simulink model "solution_1"  (R2016a)
settings: Solver=VariableStepAuto  StartTime=0.0  StopTime=10  RelTol=1e-3
undefined symbols (not defined in the file): doppler, fdesignblkfcn, gcbh, startfcn_spectrum_analyzer
libraries: commchan3 x6, dspsrcs4 x5, commrflib2 x5, commanapbnd3 x4, dspsigops x4, commdigbbndpm3 x4, commrandsrc3 x3, dspmtrx3 x1, commanabbnd3 x1, dspfdesign x1, dspspect3 x1, commutil2 x1
settings Model: Creator=Schala  LastModifiedBy=Schala

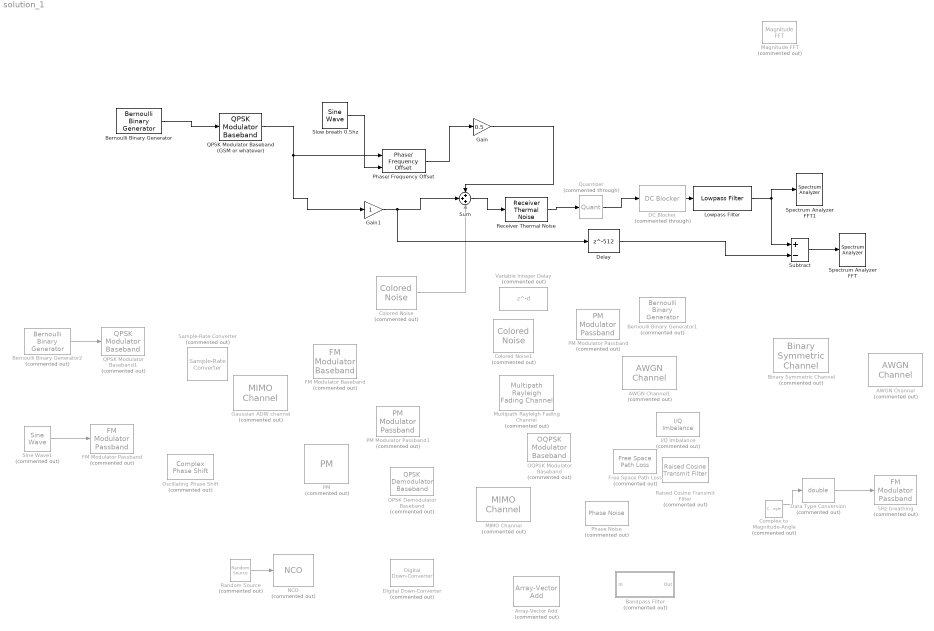
== system solution_1 ==
  "5Hz breathing " : commanapbnd3/FM Modulator Passband  Commented=on  Fc=5  Ph=0  Kc=66
  AWGN Channel : commchan3/AWGN Channel  Commented=on  InputProcessing=Columns as channels (frame based)  seed=67  noiseMode="Signal to noise ratio  (Eb/No)"  EbNodB=10  EsNodB=10  SNRdB=10  bitsPerSym=1  Ps=1  Tsym=1  variance=1
  AWGN Channel1 : commchan3/AWGN Channel  Commented=on  InputProcessing=Columns as channels (frame based)  seed=67  noiseMode="Signal to noise ratio  (Eb/No)"  EbNodB=10  EsNodB=10  SNRdB=10  bitsPerSym=1  Ps=1  Tsym=1  variance=1
  Array-Vector Add : dspmtrx3/Array-Vector Add  Commented=on  Dimension=1  V_Source=Input port  V_VectFromMask=[0.5 0.25]  firstCoeffSignedness=Auto  firstCoeffDataTypeStr=Inherit: Same word length as input  firstCoeffLastDataTypeStr=Inherit: Same word length as input  firstCoeffMin=[]  firstCoeffMax=[]  outputSignedness=Auto  outputDataTypeStr=Inherit: Same as accumulator  outputLastDataTypeStr=Inherit: Same as accumulator  outputMin=[]  outputMax=[]  accumSignedness=Auto  prodOutputSignedness=Auto  roundingMode=Floor  overflowMode=off
  Bandpass Filter : Subsystem  Commented=on  DialogController=fdesignblkfcn  InitFcn=fdesignblkfcn(gcbh, {'InitFcn'});  mask(Bandpass Filter){}
      mask help: Design a bandpass filter
      settings: CopyFcn=fdesignblkfcn(gcbh, {'CopyFcn'});
      mask Help: helpview(mapfilelocation('dsp'), 'dspbandpassfilter');
      mask Display: disp('Bandpass');
  Bernoulli Binary Generator : commrandsrc3/Bernoulli Binary Generator  ProbabilityOfZero=0.5  SeedSource=Auto  Seed=0  SampleTime=2.4e-6  SamplesPerFrame=1  OutputDataType=double  SimulateUsing=Code generation
  Bernoulli Binary Generator1 : commrandsrc3/Bernoulli Binary Generator  Commented=on  ProbabilityOfZero=0.5  SeedSource=Auto  Seed=0  SampleTime=1e-9  SamplesPerFrame=1  OutputDataType=single  SimulateUsing=Interpreted execution
  Bernoulli Binary Generator2 : commrandsrc3/Bernoulli Binary Generator  Commented=on  ProbabilityOfZero=0.5  SeedSource=Auto  Seed=0  SampleTime=2.4e-6  SamplesPerFrame=2  OutputDataType=single  SimulateUsing=Code generation
  Binary Symmetric Channel : commchan3/Binary Symmetric Channel  Commented=on  P=0.05  s=71  E=on  outDtype=double
  Colored Noise : dspsrcs4/Colored Noise  Commented=on  Color=white  InverseFrequencyPower=1  NumChannels=1  OutputDataType=single  SamplesPerFrame=1  SampleTime=2.4e-6  RandomStream=mt19937ar with seed  Seed=67  SimulateUsing=Code generation
  Colored Noise1 : dspsrcs4/Colored Noise  Commented=on  Color=white  InverseFrequencyPower=1  NumChannels=1  OutputDataType=single  SamplesPerFrame=1  SampleTime=2.4e-6  RandomStream=mt19937ar with seed  Seed=67  SimulateUsing=Code generation
  Complex to Magnitude-Angle : ComplexToMagnitudeAngle  Commented=on
  DC Blocker : dspsigops/DC Blocker  Commented=through  Algorithm=IIR  NormalizedBandwidth=0.001  Length=8  Order=6  SimulateUsing=Code generation
  Data Type Conversion : DataTypeConversion  Commented=on  OutDataTypeStr=double
  Delay : Delay  DelayLength=512  InputProcessing=Columns as channels (frame based)
  Digital Down-Converter : dspsigops/Digital Down-Converter  Commented=on  DecimationFactor=416  MinimumOrderDesign=on  NumCICSections=3  SecondFilterOrder=12  ThirdFilterOrder=10  Bandwidth=66.66666  StopbandFrequencySource=Auto  StopbandFrequency=150000  PassbandRipple=0.1  StopbandAttenuation=60  Oscillator=Sine wave  CenterFrequency=0  NumAccumulatorBits=16  NumQuantizedAccumulatorBits=12  Dither=on  NumDitherBits=4  InheritSampleRate=off  SampleRate=2.4e6  outputMin=[]  outputMax=[]  SimulateUsing=Code generation
  FM Modulator Baseband : commanabbnd3/FM Modulator Baseband  Commented=on  FrequencyDeviation=67  SimulateUsing=Code generation
  FM Modulator Passband : commanapbnd3/FM Modulator Passband  Commented=on  Fc=1e9  Ph=0  Kc=1
  Free Space Path Loss : commrflib2/Free Space Path Loss  Commented=on  mode=Decibels  dB=10  d=0.100  fc=1920
  Gain : Gain  Gain=0.5  OutDataTypeStr=double
  Gain1 : Gain  OutDataTypeStr=double
  Gaussian ADW channel : commchan3/MIMO Channel  Commented=on  SampleRate=240000  PathDelays=0  AveragePathGains=-40  NormalizePathGains=off  FadingDistribution=Rayleigh  KFactor=3  DirectPathDopplerShift=0  DirectPathInitialPhase=0  MaximumDopplerShift=66.6666  DopplerSpectrum=doppler( 'Jakes' )  SpatialCorrelation=off  NumTransmitAntennas=1  NumReceiveAntennas=1  TransmitCorrelationMatrix=[1 0; 0 1]  ReceiveCorrelationMatrix=[1 0; 0 1]  AntennaSelection=Off  NormalizeChannelOutputs=on  FadingTechnique=Filtered Gaussian noise  NumSinusoids=48  InitialTimeSource=Property  InitialTime=0  RandomStream=mt19937ar with seed  Seed=73  PathGainsOutputPort=off  Visualization=Doppler spectrum  AntennaPairsToDisplay=[ 1, 1 ]  PathsForDopplerDisplay=1  SamplesToDisplay=25%  SimulateUsing=Interpreted execution
  I/Q Imbalance : commrflib2/I//Q Imbalance  Commented=on  ampImbal=0  phsImbal=0  Idc=0  Qdc=0
  Lowpass Filter : dspfdesign/Lowpass Filter  FilterType=IIR  DesignForMinimumOrder=on  FilterOrder=50  PassbandFrequency=300  StopbandFrequency=1.19e6  PassbandRipple=0.1  StopbandAttenuation=80  InheritSampleRate=off  SampleRate=2.4e6  roundingMode=Floor  coeffsDataTypeStr=fixdt(1,16)  SimulateUsing=Code generation
  MIMO Channel : commchan3/MIMO Channel  Commented=on  SampleRate=1  PathDelays=0  AveragePathGains=0  NormalizePathGains=on  FadingDistribution=Rayleigh  KFactor=3  DirectPathDopplerShift=0  DirectPathInitialPhase=0  MaximumDopplerShift=0.001  DopplerSpectrum=doppler( 'Jakes' )  SpatialCorrelation=off  NumTransmitAntennas=2  NumReceiveAntennas=2  TransmitCorrelationMatrix=[1 0; 0 1]  ReceiveCorrelationMatrix=[1 0; 0 1]  AntennaSelection=Off  NormalizeChannelOutputs=on  FadingTechnique=Filtered Gaussian noise  NumSinusoids=48  InitialTimeSource=Property  InitialTime=0  RandomStream=mt19937ar with seed  Seed=73  PathGainsOutputPort=off  Visualization=Off  AntennaPairsToDisplay=[ 1, 1 ]  PathsForDopplerDisplay=1  SamplesToDisplay=25%  SimulateUsing=Interpreted execution
  Magnitude FFT : dspspect3/Magnitude FFT  Commented=on  mag_or_magsq=Magnitude squared  FFTImplementation=Auto  fftLenInherit=off  fftsize=36120  WrapInput=off
  Multipath Rayleigh Fading Channel : commchan3/Multipath Rayleigh Fading Channel  Commented=on  maxDopplerShift=40  spectrumType=Jakes  sigmaGaussian=1/sqrt(2)  coeffRounded=[1 -1.72 0.785]  freqMinMaxRJakes=[0 1]  freqMinMaxAJakes=[0 1]  sigmaGaussian1=1/sqrt(2)  sigmaGaussian2=1/sqrt(2)  centerFreqGaussian1=0.0  centerFreqGaussian2=0.0  gainGaussian1=0.5  gainGaussian2=0.5  coeffBell=9  dopplerSpectrum=doppler.jakes  pathDelays=[0 2e-6]  avgPathGaindB=[0 -3]  normalizePathGains=on  seed=73  enableProbe=0  openVisAtStart=off  outPathGains=off  outDelay=off
  NCO : dspsigops/NCO  Commented=on  AccIncSrc=Specify via dialog  AccInc=628  PhaseOffsetSrc=Input port  PhaseOffset=0  AccumWL=16  HasDither=off  DitherWL=4  PNgeneratorLength=19  HasPhaseQuantizer=off  TableDepth=12  HasOutputPhaseError=off  Formula=Complex exponential  DataType=single  OutputWL=16  OutputFL=14  CompMethod=Table lookup (no interpolation)  SampleTime=1  SamplesPerFrame=1  OutputFrames=off
  OQPSK Modulator Baseband : commdigbbndpm3/OQPSK Modulator Baseband  Commented=on  InType=Integer  Ph=0  RateOptions=Enforce single-rate processing  outDtype=double  outUDDataType=sfix(16)  outWordLen=16  outFracLenMode=Best precision  outFracLen=15  outDataTypeStr=double  outLastDataTypeStr=double
  Oscillating Phase Shift : commutil2/Complex Phase Shift  Commented=on
  PM : commhdlmod/PM  Commented=on
  PM Modulator Passband : commanapbnd3/PM Modulator Passband  Commented=on  Fc=2.4e6  Ph=0  Kc=pi/2
  PM Modulator Passband1 : commanapbnd3/PM Modulator Passband  Commented=on  Fc=300  Ph=0  Kc=pi/2
  Phase Noise : commrflib2/Phase Noise  Commented=on  PhNs=[-60]  Fo=[20]  Fs=2400000  seed=2137
  Phase/ Frequency Offset : commrflib2/Phase// Frequency Offset  phaseOffset=0  freqPort=on  freqOffset=67
  QPSK Demodulator Baseband : commdigbbndpm3/QPSK Demodulator Baseband  Commented=on  OutType=Integer  DecType=Hard decision  VarSource=Dialog  Variance=1  Dec=Gray  Ph=pi/4  outDtype1=Inherit via internal rule  outDtype2=Inherit via internal rule  derotateFactorWordLen=16  derotateFactorDataTypeStr=Inherit: Same word length as input  derotateFactorLastDataTypeStr=Inherit: Same word length as input
  QPSK Modulator Baseband (GSM or whatever) : commdigbbndpm3/QPSK Modulator Baseband  InType=Integer  Enc=Gray  Ph=pi/4  outDtype=double  outWordLen=16  outUDDataType=sfix(16)  outFracLenMode=Best precision  outFracLen=15  outDataTypeStr=double  outLastDataTypeStr=double
  QPSK Modulator Baseband1 : commdigbbndpm3/QPSK Modulator Baseband  Commented=on  InType=Bit  Enc=Gray  Ph=pi/4  outDtype=single  outWordLen=16  outUDDataType=sfix(16)  outFracLenMode=Best precision  outFracLen=15  outDataTypeStr=single  outLastDataTypeStr=single
  Quantizer : Quantizer  Commented=through  LinearizeAsGain=off
  Raised Cosine Transmit Filter : commfilt2/Raised Cosine Transmit Filter  Commented=on  filtType=Square root  R=0.2  filtSpan=10  N=8  filterGain=1  RateOptions=Allow multirate processing  framing=Mute  checkCoeff=off  variableName=rcTxFilt  checkGain=Normalized  sampMode=Mute  saveAsFlag=0  currentFiltSpan=10  D=5  launchFVT=on  roundingMode=Floor  overflowMode=off  coeffDataTypeStr=Inherit: Same word length as input  coeffMin=[]  coeffMax=[]  coeffLastDataTypeStr=Inherit: Same word length as input  outputDataTypeStr=Inherit: Same as accumulator  outputMin=[]  outputMax=[]  outputLastDataTypeStr=Inherit: Same as accumulator
  Random Source : dspsrcs4/Random Source  Commented=on  SrcType=Uniform  NormMethod=Ziggurat  CltLength=12  MinVal=-3.14  MaxVal=3.14  MeanVal=0  VarVal=1  RepMode=Not repeatable  rawSeed=1  IsInherit=off  SampMode=Discrete  SampTime=2.4e-6  SampFrame=416  DataType=Double  OutComplex=Real  OutputFrames=off
  Receiver Thermal Noise : commrflib2/Receiver Thermal Noise  method=Noise temperature  ntemp=290  nfigure=3.01  nfactor=2  seed=67987
  Sample-Rate Converter : dspsigops/Sample-Rate Converter  Commented=on  InputSampleRate=9.984e8  OutputSampleRate=2.4e6  OutputRateTolerance=0  Bandwidth=134  StopbandAttenuation=80  SimulateUsing=Code generation
  Sine Wave1 : dspsrcs4/Sine Wave  Commented=on  Amplitude=1  Frequency=1e9  Phase=0  SampleMode=Discrete  OutComplex=Real  CompMethod=Trigonometric fcn  TableSize=Speed  SampleTime=2e9  SamplesPerFrame=832  ResetState=Restart at time zero  OutputFrames=off  dataType=single  wordLen=16  udDataType=sfix(16)  fracBitsMode=Best precision  numFracBits=15  OutDataTypeStr=single  LastOutDataTypeStr=single
  Slow breath 0.5hz : dspsrcs4/Sine Wave  Amplitude=67  Frequency=0.5  Phase=0  SampleMode=Discrete  OutComplex=Real  CompMethod=Trigonometric fcn  TableSize=Speed  SampleTime=2.4e-6  SamplesPerFrame=1  ResetState=Restart at time zero  OutputFrames=off  dataType=double  wordLen=16  udDataType=sfix(16)  fracBitsMode=Best precision  numFracBits=15  OutDataTypeStr=double  LastOutDataTypeStr=double
  Spectrum Analyzer FFT : SpectrumAnalyzer  StartFcn=startfcn_spectrum_analyzer;
  Spectrum Analyzer FFT1 : SpectrumAnalyzer  StartFcn=startfcn_spectrum_analyzer;
  Subtract : Sum  Inputs=+-
  Sum : Sum  Inputs=+++  InputSameDT=on
  Variable Integer Delay : Delay  Commented=on  DelayLengthSource=Input port  InputProcessing=Columns as channels (frame based)
      settings: InputPortMap=u0,p1
  wires:
  Random Source/1 -> NCO/1
  Bernoulli Binary Generator/1 -> QPSK Modulator Baseband (GSM or whatever)/1
  Gain/1 -> Sum/1
  Colored Noise/1 -> Sum/3
  Sum/1 -> Receiver Thermal Noise/1
  Lowpass Filter/1 -> Subtract/1, Spectrum Analyzer FFT1/1
  Subtract/1 -> Spectrum Analyzer FFT/1
  Bernoulli Binary Generator2/1 -> QPSK Modulator Baseband1/1
  Data Type Conversion/1 -> "5Hz breathing "/1
  Complex to Magnitude-Angle/1 -> Data Type Conversion/1
  DC Blocker/1 -> Lowpass Filter/1
  Receiver Thermal Noise/1 -> Quantizer/1
  Quantizer/1 -> DC Blocker/1
  Phase/ Frequency Offset/1 -> Gain/1
  Slow breath 0.5hz/1 -> Phase/ Frequency Offset/2
  Sine Wave1/1 -> FM Modulator Passband/1
  QPSK Modulator Baseband (GSM or whatever)/1 -> Phase/ Frequency Offset/1, Gain1/1
  Gain1/1 -> Delay/1, Sum/2
  Delay/1 -> Subtract/2

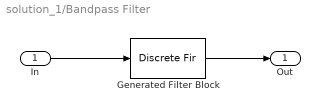
== system solution_1/Bandpass Filter ==
  In : Inport
  Generated Filter Block : DiscreteFir  Tag=BlockMethodSubSystem  Coefficients=[-0.0008992291487744296 0.0016414518747943749 0.0031352071842225397 -0.0040707550828814922 -0.0063731852227904111 0.0074874286806090491 0.0098354319566295711 -0.010189316513446216 -0.011302794465874122 0.0096929185841818435 0.0079428653987464216 -0.0031368247881221642 0.0028299878877943137 -0.011508674243001471 -0.022080136219461581 0.034245325424507672 0.048356661648905473 -0.062355369169884239 -0.077503478162593897 0.090687768153125653 0.10353171105844157 -0.11297860084229834 -0.12035866024978455 0.12379360801539134 0.12379360801539134 -0.12035866024978455 -0.11297860084229834 0.10353171105844157 0.090687768153125653 -0.077503478162593897 -0.062355369169884239 0.048356661648905473 0.034245325424507672 -0.022080136219461581 -0.011508674243001471 0.0028299878877943137 -0.0031368247881221642 0.0079428653987464216 0.0096929185841818435 -0.011302794465874122 -0.010189316513446216 0.0098354319566295711 0.0074874286806090491 -0.0063731852227904111 -0.0040707550828814922 0.0031352071842225397 0.0016414518747943749 -0.0008992291487744296]  InputProcessing=Columns as channels (frame based)
  Out : Outport
  wires:
  In/1 -> Generated Filter Block/1
  Generated Filter Block/1 -> Out/1
